simulink model "BAT_th"  (R2018b)
settings: Solver=ode15s  StartTime=0.0  StopTime=simTime  MaxStep=0.1  RelTol=1e-3
values from neighbouring files (symbols this model uses):
  iniPos = [xOffset*(0:NumSys-1); operZ*ones(1,NumSys)].*ones(2,NumSys)    [BAT_ts.m]
  maxWinch = 0.5    [BAT_ts.m]
undefined symbols (not defined in the file or in its folder): SP
libraries: flowInterp_ul x1, planarBATctrllr_ul x1, BAT_cl x1
settings Model: Creator=Ayaz  LastModifiedBy=Ayaz

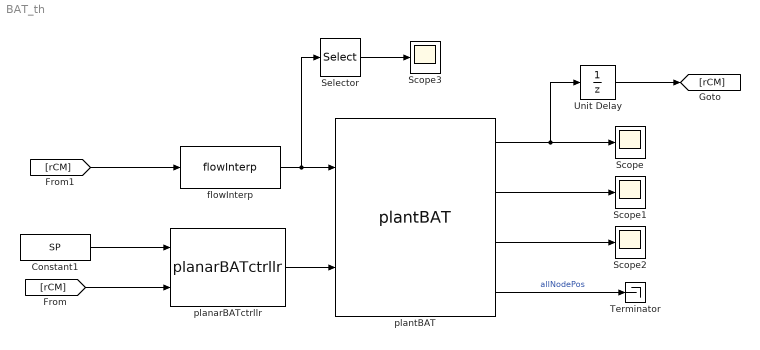
== system BAT_th ==
  Constant1 : Constant  Value=SP  VectorParams1D=off
  Scope{,1..3} (4 alike) : Scope
  Selector : Selector  NumberOfDimensions=2  InputPortWidth=3  IndexOptions=Index vector (dialog),Select all  Indices=1,1  OutputSizes=1,1
  Terminator : Terminator
  Unit Delay : UnitDelay  InitialCondition=iniPos  SampleTime=-1
  flowInterp : flowInterp_ul/flowInterp  altiVals=heights  flowVals=Flows
  planarBATctrllr : planarBATctrllr_ul/planarBATctrllr  kp=kp  kd=kd  tau=tau
  plantBAT : BAT_cl/plantBAT  rhoF=rhoFluid  gravAcc=gravAcc  mT=mass  BF=BF  Sref=Sref  Cd=dragCoeff  numNode=numNode  tetDia=tetDia  tetDensity=tetRho  tetCD=tetCD  tetYoungs=tetYoungs  tetZeta=tetZeta  ini_rCM=iniPos  ini_vCM=iniVel  gndNodePos=gndNodePos  iniLength=iniTetherLength  maxRelease=maxWinch  maxTug=-maxWinch
  wires:
  plantBAT/1 -> Unit Delay/1, Scope/1
  plantBAT/2 -> Scope1/1
  plantBAT/3 -> Scope2/1
  plantBAT/4 -> Terminator/1  "allNodePos"
  planarBATctrllr/1 -> plantBAT/2
  [rCM] -> planarBATctrllr/2
  Constant1/1 -> planarBATctrllr/1
  [rCM] -> flowInterp/1
  flowInterp/1 -> Selector/1, plantBAT/1
  Unit Delay/1 -> [rCM]
  Selector/1 -> Scope3/1
